simulink model "FSM_parking_gate_v4"  (R2024a)
settings: Solver=FixedStepAuto  StartTime=0.0  StopTime=100  FixedStep=0.2  RelTol=1e-3
settings Model: PacingRate=2  Creator=ArriGE66  LastModifiedBy=Bocchio
settings ModelReferenceCC: EnableRefExpFcnMdlSchedulingChecks=on
settings RTWCC: GPUComputeCapability=3.5

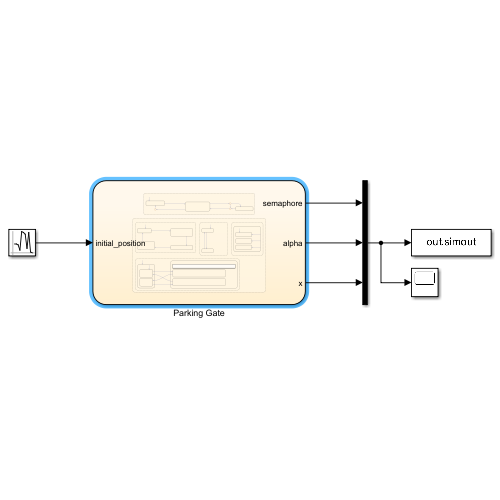
[thumbnail: Simulink's stored preview of the top-level diagram]
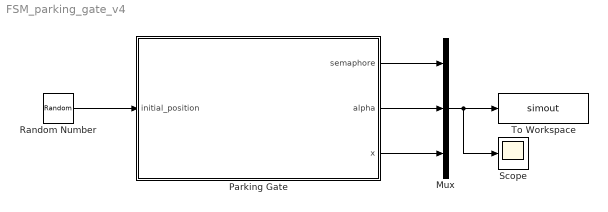
== system FSM_parking_gate_v4 ==
  Mux : Mux  Inputs=3
  Parking Gate : Stateflow chart  TreatAsAtomicUnit=on
  Random Number : RandomNumber  Mean=-15  Variance=5  SampleTime=0.2
  Scope : Scope
  To Workspace : ToWorkspace  VariableName=simout  SampleTime=-1
  wires:
  Random Number/1 -> Parking Gate/1(initial_position)
  Mux/1 -> To Workspace/1, Scope/1
  Parking Gate/1(semaphore) -> Mux/1
  Parking Gate/2(alpha) -> Mux/2
  Parking Gate/3(x) -> Mux/3

== stateflow chart FSM_parking_gate_v4/Parking Gate ==
  state Vehicle [parallel]
    settings: executionOrder=1
    state Spawning
      entry: x = initial_position;
    state Driving
      during:
      v = min(abs(x), 30/3.6)  + 10e-2;
      x = min(x + v*dt, checkpoint);
    state Waiting
      entry: send(TicketPayed)
    (default) -> Spawning
    Driving -> (junction 287) [order 1] : [x == checkpoint]
    (junction 287) -> Waiting [order 1] : [semaphore == 1]
    Spawning -> Driving : {checkpoint = gate_pos;}
    (junction 287) -> (junction 286) [order 2]
    (junction 278) -> Spawning : after(10, sec)
    (junction 286) -> Driving : [semaphore == 3]
        | {checkpoint = +inf;}
    Waiting -> (junction 286)
    Driving -> (junction 278) [order 2] : [in(ParkingGate.Gate.Idling.GateDown)]
  state ParkingGate [parallel]
    settings: executionOrder=2
    state Semaphore [parallel]
      settings: executionOrder=2
      state On
        state Red
          entry: semaphore = 1;
        state Yellow
          entry: semaphore = 2;
        state Green
          entry: semaphore = 3;
        (default) -> Red
        On -> Red [order 1] : Red
        On -> Yellow [order 2] : Yellow
        On -> Green [order 3] : Green
    state Controller [parallel]
      settings: executionOrder=1
      state Idling
      state GateOpening
        entry:
        send(Yellow, Semaphore)
        send(Raise, Gate)
      state GateClosing
        entry:
        send(Lower, Gate)
        send(Red, Semaphore)
      state WaitingClearance
        entry: send(Green, Semaphore)
      (default) -> ParkingGate.Controller.Idling
      ParkingGate.Controller.Idling -> GateOpening : TicketPayed
      GateClosing -> ParkingGate.Controller.Idling : [in(Gate.Idling.GateDown)]
      GateOpening -> WaitingClearance : [in(Gate.Idling.GateUp)]
      WaitingClearance -> GateClosing : [in(PhotoCell.Free)]
    state PhotoCell [parallel]
      settings: executionOrder=3
      state Free
      state Occupied
      (default) -> Free
      Occupied -> Free : [
          |   x<=(gate_x - 50e-2) || ...
          |   x>=(gate_x + car_length)
          | ]
      Free -> Occupied : [
          |   x>(gate_x - 50e-2) && ...
          |   x<(gate_x + car_length)
          | ]
    state Gate [parallel]
      settings: executionOrder=4
      state Moving
        state Raising
          entry: [time, alphas] = computeTrapezoidalProfile(alpha, 90, max_omega, max_omega_dot);
          during: alpha = interp1(time, alphas, elapsed(sec), 'nearest', 'extrap');
        state Lowering
          entry: [time, alphas] = computeTrapezoidalProfile(alpha, 0, max_omega, max_omega_dot);
          during: alpha = interp1(time, alphas, elapsed(sec), 'nearest', 'extrap');
      state Idling
        state GateDown
          entry: alpha = 0;
        state GateUp
          entry: alpha = 90;
        (default) -> GateDown
      (default) -> ParkingGate.Gate.Idling
      GateDown -> Raising : Raise
      Raising -> GateUp : [alpha == 90]
      Lowering -> GateDown : [alpha == 0]
      GateUp -> Lowering : Lower
  data: pos_current function_input; pos_target function_input; max_vel function_input; max_acc function_input; t_vec function_output; x_vec function_output; max_omega_dot constant double =1; max_omega constant double =4; car_length constant double =3; gate_x constant double =0; time local double; alphas local; semaphore output; alpha output; gate_up local; initial_position input; checkpoint local; v local; dt constant double =0.2; gate_pos constant double =0; x output double
  events: Raise local FUNCTION_CALL_EVENT; Lower local FUNCTION_CALL_EVENT; Red local FUNCTION_CALL_EVENT; Yellow local FUNCTION_CALL_EVENT; Green local FUNCTION_CALL_EVENT; TicketPayed local FUNCTION_CALL_EVENT
  function [t_vec, x_vec] = computeTrapezoidalProfile(pos_current, pos_target, max_vel, max_acc):
    | function [t_vec, x_vec] = computeTrapezoidalProfile(pos_current, pos_target, max_vel, max_acc)
    | % COMPUTE_TRAPEZOIDAL_PROFILE Generates time and angle points for a trapezoidal profile
    | % At first checks if a trapezoidal profile is feasible or is necessary to
    | % fallback to a triangular one.
    | 
    | delta_pos = pos_target - pos_current;
    | time_acc_phase = max_vel / max_acc;
    | delta_pos_acc_phase = 0.5 * max_acc * time_acc_phase^2;
    | 
    | if 2 * delta_pos_acc_phase < abs(delta_pos)
    |     % Trapezoidal profile
    |     t1 = time_acc_phase;
    |     t2 = (abs(delta_pos) - 2 * delta_pos_acc_phase) / max_vel;
    |     t3 = time_acc_phase;
    | else
    |     % Triangular profile
    |     max_vel = sqrt(abs(delta_pos) * max_acc);
    |     t1 = max_vel / max_acc;
    |     t2 = 0;
    |     t3 = max_vel / max_acc;
    | end
    | 
    | 
    | % Trapezoidal profile template (HP: s0 = 0, v0 = 0)
    | acc = max_acc * sign(delta_pos);
    | vel = max_vel * sign(delta_pos);
    | profile_template = @(t) ...
    |     (t <= t1) .*                             (1/2 * acc * t.^2) + ...
    |     (t > t1 & t <= (t1 + t2)) .*             (1/2 * acc * t1^2 + vel * (t - t1)) + ...
    |     (t > (t1 + t2) & t <= (t1 + t2 + t3)) .* (1/2 * acc * t1^2 + vel * t2 + vel * (t - (t2 + t1)) - 1/2 * acc * (t - (t1 + t2)).^2) + ...
    |     (t > (t1 + t2 + t3)) .*                  (1/2 * acc * t1^2 + vel * t2 + vel * t3 - 1/2 * acc * t3.^2);
    | 
    | % Profile generation
    | t_vec = linspace(0, t1 + t2 + t3, 100);
    | x_vec = profile_template(t_vec) + pos_current;
    | 
    | end
